simulink model "Ref49_ICAS_compare"  (R2025b)
settings: Solver=ode4  StartTime=0.0  StopTime=20  FixedStep=0.001  RelTol=1e-3
settings Model: Creator=31586  LastModifiedBy=31586

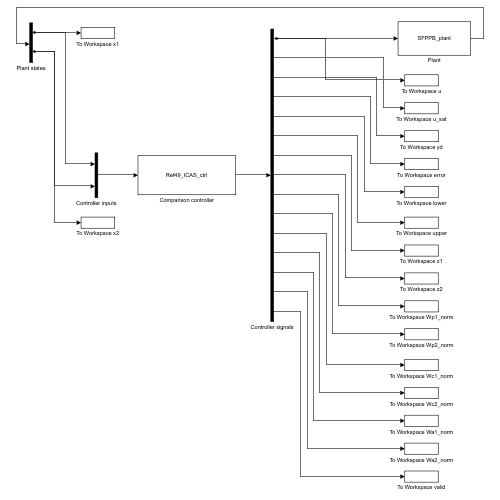
[thumbnail: Simulink's stored preview of the top-level diagram]
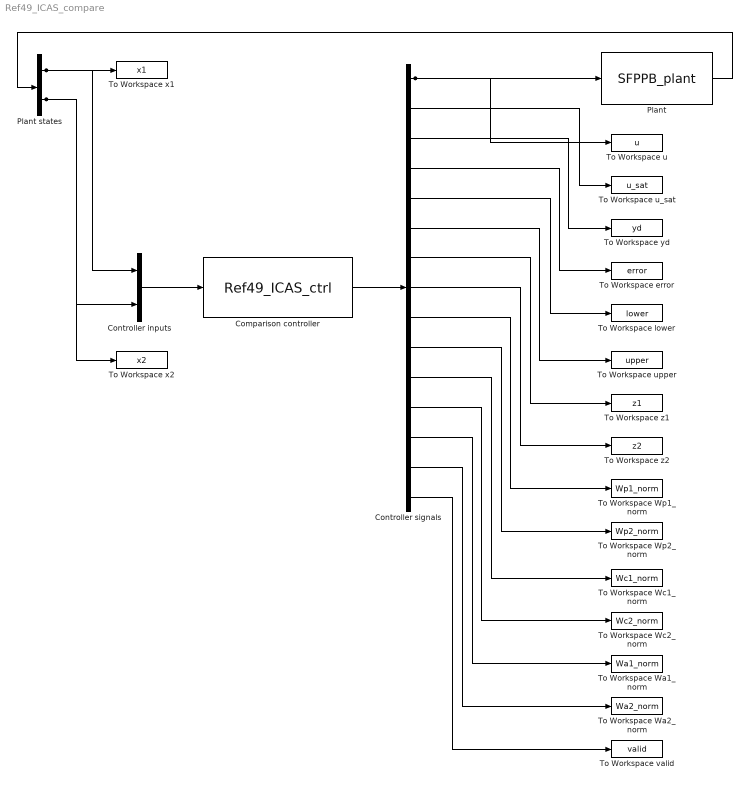
== system Ref49_ICAS_compare ==
  Comparison controller : S-Function  FunctionName=Ref49_ICAS_ctrl  SFunctionDeploymentMode=off  EnableBusSupport=off
  Controller inputs : Mux  Inputs=2
  Controller signals : Demux  Outputs=15
  Plant : S-Function  FunctionName=SFPPB_plant  SFunctionDeploymentMode=off  EnableBusSupport=off
  Plant states : Demux  Outputs=2
  To Workspace Wa1_norm : ToWorkspace  VariableName=Wa1_norm  SaveFormat=Timeseries  SampleTime=-1
  To Workspace Wa2_norm : ToWorkspace  VariableName=Wa2_norm  SaveFormat=Timeseries  SampleTime=-1
  To Workspace Wc1_norm : ToWorkspace  VariableName=Wc1_norm  SaveFormat=Timeseries  SampleTime=-1
  To Workspace Wc2_norm : ToWorkspace  VariableName=Wc2_norm  SaveFormat=Timeseries  SampleTime=-1
  To Workspace Wp1_norm : ToWorkspace  VariableName=Wp1_norm  SaveFormat=Timeseries  SampleTime=-1
  To Workspace Wp2_norm : ToWorkspace  VariableName=Wp2_norm  SaveFormat=Timeseries  SampleTime=-1
  To Workspace error : ToWorkspace  VariableName=error  SaveFormat=Timeseries  SampleTime=-1
  To Workspace lower : ToWorkspace  VariableName=lower  SaveFormat=Timeseries  SampleTime=-1
  To Workspace u : ToWorkspace  VariableName=u  SaveFormat=Timeseries  SampleTime=-1
  To Workspace u_sat : ToWorkspace  VariableName=u_sat  SaveFormat=Timeseries  SampleTime=-1
  To Workspace upper : ToWorkspace  VariableName=upper  SaveFormat=Timeseries  SampleTime=-1
  To Workspace valid : ToWorkspace  VariableName=valid  SaveFormat=Timeseries  SampleTime=-1
  To Workspace x1 : ToWorkspace  VariableName=x1  SaveFormat=Timeseries  SampleTime=-1
  To Workspace x2 : ToWorkspace  VariableName=x2  SaveFormat=Timeseries  SampleTime=-1
  To Workspace yd : ToWorkspace  VariableName=yd  SaveFormat=Timeseries  SampleTime=-1
  To Workspace z1 : ToWorkspace  VariableName=z1  SaveFormat=Timeseries  SampleTime=-1
  To Workspace z2 : ToWorkspace  VariableName=z2  SaveFormat=Timeseries  SampleTime=-1
  wires:
  Plant states/2 -> Controller inputs/2, To Workspace x2/1
  Plant states/1 -> Controller inputs/1, To Workspace x1/1
  Controller inputs/1 -> Comparison controller/1
  Comparison controller/1 -> Controller signals/1
  Controller signals/1 -> Plant/1, To Workspace u/1
  Controller signals/3 -> To Workspace yd/1
  Controller signals/2 -> To Workspace u_sat/1
  Controller signals/10 -> To Workspace Wp2_norm/1
  Controller signals/8 -> To Workspace z2/1
  Controller signals/6 -> To Workspace upper/1
  Controller signals/4 -> To Workspace error/1
  Controller signals/11 -> To Workspace Wc1_norm/1
  Controller signals/9 -> To Workspace Wp1_norm/1
  Controller signals/7 -> To Workspace z1/1
  Controller signals/5 -> To Workspace lower/1
  Controller signals/12 -> To Workspace Wc2_norm/1
  Controller signals/13 -> To Workspace Wa1_norm/1
  Controller signals/14 -> To Workspace Wa2_norm/1
  Controller signals/15 -> To Workspace valid/1
  Plant/1 -> Plant states/1
